simulink model "simulation"  (R2021a)
settings: Solver=VariableStepAuto  StartTime=0.0  StopTime=1  RelTol=1e-3
values from neighbouring files (symbols this model uses):
  b = 2.9e-05    [Prametre.m]
  d = 3.23e-07    [Prametre.m]
  g = 9.81    [Prametre.m]
  Ix = 0.0075    [Prametre.m]
  Iy = 0.0075    [Prametre.m]
  Iz = 0.013    [Prametre.m]
  Jr = 2.83e-05    [Prametre.m]
  K1 = 5.57e-04    (= 0.000557)    [Prametre.m]
  K2 = 5.57e-04    (= 0.000557)    [Prametre.m]
  K3 = 6.35e-04    (= 0.000635)    [Prametre.m]
  K4 = 5.57e-04    (= 0.000557)    [Prametre.m]
  K5 = 5.57e-04    (= 0.000557)    [Prametre.m]
  K6 = 6.35e-04    (= 0.000635)    [Prametre.m]
  l = 0.23    [Prametre.m]
  m = 0.65    [Prametre.m]
libraries: pid_lib x1
settings Model: Creator=dell  LastModifiedBy=Copytop
settings SolverCC: AlgebraicLoopSolver=TrustRegion
settings DataIOCC: ReturnWorkspaceOutputs=off
settings DebuggingCC: SFMachineParentedDataDiag=warning  ArithmeticOperatorsInVariantConditions=warning
settings SFSimCC: SimUseLocalCustomCode=off  CustomCodeUndefinedFunction=UseInterfaceOnly
settings RTWCC: RTWUseLocalCustomCode=off
settings CodeAppCC: StateflowObjectComments=on
settings SimscapeCC: SimscapeNormalizeSystem=off

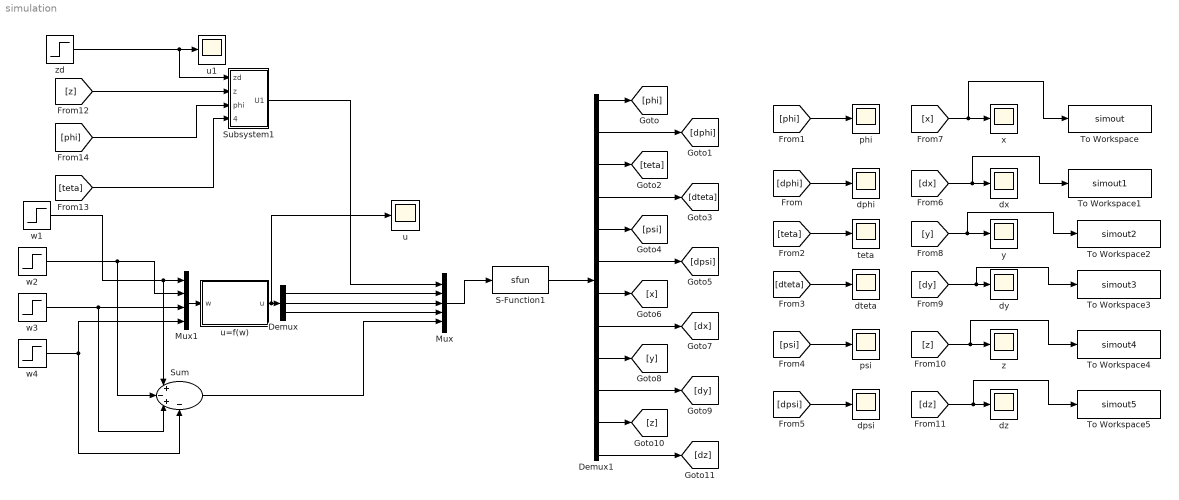
== system simulation ==
  Demux : Demux  Outputs=3
  Demux1 : Demux  Outputs=12
  Mux : Mux  Inputs=5
  Mux1 : Mux
  S-Function1 : S-Function  FunctionName=sfun  Parameters=m;l;Ix;Iy;Iz;Jr;b;d;K1;K2;K3;K4;K5;K6;g  SFunctionDeploymentMode=off  EnableBusSupport=off
  Subsystem1 : Subsystem
  Sum : Sum  Inputs=|+-+-
  To Workspace : ToWorkspace  VariableName=simout  SaveFormat=Timeseries  SampleTime=-1
  To Workspace1 : ToWorkspace  VariableName=simout1  SaveFormat=Timeseries  SampleTime=-1
  To Workspace2 : ToWorkspace  VariableName=simout2  SaveFormat=Timeseries  SampleTime=-1
  To Workspace3 : ToWorkspace  VariableName=simout3  SaveFormat=Timeseries  SampleTime=-1
  To Workspace4 : ToWorkspace  VariableName=simout4  SaveFormat=Timeseries  SampleTime=-1
  To Workspace5 : ToWorkspace  VariableName=simout5  SaveFormat=Timeseries  SampleTime=-1
  dphi : Scope
  dpsi : Scope
  dteta : Scope
  dx : Scope
  dy : Scope
  dz : Scope
  phi : Scope
  psi : Scope
  teta : Scope
  u : Scope
  u1 : Scope
  u=f(w) : MATLAB Function  TreatAsAtomicUnit=on
  w{1..4} (4 alike) : Step  Time=0  After=200  SampleTime=0
  x : Scope
  y : Scope
  z : Scope
  zd : Step  Time=0  Before=5  After=5  SampleTime=0
  wires:
  Mux/1 -> S-Function1/1
  w2/1 -> Sum/2, Mux1/2
  Mux1/1 -> u=f(w)/1(w)
  w3/1 -> Sum/3, Mux1/3
  w4/1 -> Mux1/4, Sum/4
  u=f(w)/1(u) -> u/1, Demux/1
  S-Function1/1 -> Demux1/1
  Demux1/1 -> [phi]
  Demux1/3 -> [teta]
  Demux1/5 -> [psi]
  Demux1/7 -> [x]
  Demux1/9 -> [y]
  Demux1/11 -> [z]
  [phi] -> phi/1
  [dphi] -> dphi/1
  [teta] -> teta/1
  [dteta] -> dteta/1
  [psi] -> psi/1
  [dpsi] -> dpsi/1
  [dx] -> To Workspace1/1, dx/1
  [y] -> To Workspace2/1, y/1
  [dy] -> To Workspace3/1, dy/1
  [z] -> To Workspace4/1, z/1
  [dz] -> To Workspace5/1, dz/1
  Sum/1 -> Mux/5
  Demux1/2 -> [dphi]
  Demux1/4 -> [dteta]
  Demux1/6 -> [dpsi]
  Demux1/8 -> [dx]
  Demux1/10 -> [dy]
  Demux1/12 -> [dz]
  [z] -> Subsystem1/2(z)
  [phi] -> Subsystem1/3(phi)
  zd/1 -> Subsystem1/1(zd), u1/1
  [teta] -> Subsystem1/4(teta)
  Subsystem1/1(U1) -> Mux/1
  w1/1 -> Sum/1, Mux1/1
  Demux/1 -> Mux/2
  Demux/2 -> Mux/3
  Demux/3 -> Mux/4
  [x] -> To Workspace/1, x/1

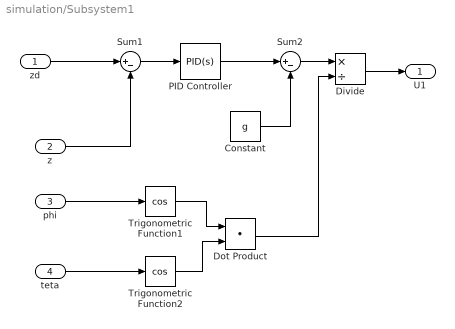
== system simulation/Subsystem1 ==
  zd : Inport
  z : Inport  Port=2
  phi : Inport  Port=3
  teta : Inport  Port=4
  Constant : Constant  Value=g
  Divide : Product  Inputs=*/
  Dot Product : DotProduct  InputSameDT=on  OutDataTypeStr=Inherit: Inherit via internal rule
  PID Controller : pid_lib/PID Controller  Controller=PID  Form=Parallel  TimeDomain=Continuous-time  UseExternalTs=off  SampleTime=-1  IntegratorMethod=Forward Euler  FilterMethod=Forward Euler  ControllerParametersSource=internal  P=100  I=0  D=42  UseFilter=on  N=100  TunerSelectOption=Transfer Function Based (PID Tuner App)  InitialConditionSource=internal  InitialConditionForIntegrator=0  InitialConditionForFilter=0  DifferentiatorICPrevScaledInput=0  ExternalReset=none  TrackingMode=off  Kt=1  LimitOutput=off  SatLimitsSource=internal  UpperSaturationLimit=inf  LowerSaturationLimit=-inf  LinearizeAsGain=on  AntiWindupMode=none  Kb=1  POutMin=[]  POutMax=[]  IOutMin=[]  IOutMax=[]  DOutMin=[]  DOutMax=[]  NOutMin=[]  NOutMax=[]  SumOutMin=[]  SumOutMax=[]  SaturationOutMin=[]  SaturationOutMax=[]  PParamMin=[]  PParamMax=[]  IParamMin=[]  IParamMax=[]  DParamMin=[]  DParamMax=[]  NParamMin=[]  NParamMax=[]  KbParamMin=[]  KbParamMax=[]  KtParamMin=[]  KtParamMax=[]  KbOutMin=[]  KbOutMax=[]  KtOutMin=[]  KtOutMax=[]  IntegratorOutMin=[]  IntegratorOutMax=[]  FilterOutMin=[]  FilterOutMax=[]  SumI1OutMin=[]  SumI1OutMax=[]  SumI2OutMin=[]  SumI2OutMax=[]  SumI3OutMin=[]  SumI3OutMax=[]  SumI4OutMin=[]  SumI4OutMax=[]  SumDOutMin=[]  SumDOutMax=[]  DifferentiatorOutMin=[]  DifferentiatorOutMax=[]  FilterDiffOutCoefMin=[]  FilterDiffOutCoefMax=[]  ReciprocalOutMin=[]  ReciprocalOutMax=[]  SumDenOutMin=[]  SumDenOutMax=[]  SumNumOutMin=[]  SumNumOutMax=[]  DivideOutMin=[]  DivideOutMax=[]  UdiffTsProdOutMin=[]  UdiffTsProdOutMax=[]  NTsProdOutMin=[]  NTsProdOutMax=[]  UintegralTsProdOutMin=[]  UintegralTsProdOutMax=[]  UngainTsProdOutMin=[]  UngainTsProdOutMax=[]  IntegratorContinuousStateAttributes=''  IntegratorStateMustResolveToSignalObject=off  IntegratorRTWStateStorageClass=Auto  FilterContinuousStateAttributes=''  FilterStateMustResolveToSignalObject=off  FilterRTWStateStorageClass=Auto  ParallelPVariant=InternalParameters  IdealPVariant=Disabled  IVariant=InternalParameters  DVariant=InternalParameters  IntegratorVariant=Continuous  SatVariant=Disabled  AWVariant=Passthrough  PCopyVariant=Disabled  TRVariant=Disabled  FdbkBlocksVariant=Forward  IdealPFdbkVariant=Disabled  SatFdbkVariant=Disabled  DerivativeFilterVariant=ContFilter  NVariant=InternalParameters  NCopyVariant=Disabled  FilterICVariant=InternalICsFilter  IntegratorICVariant=InternalICs  ExternalResetVariant=Disabled  TRSumVariant=Passthrough  SumFdbkVariant=Disabled  SumVariant=Sum_PID  TsampFilterVariant=InternalTs  TsampNgainVariant=Passthrough  TsampIntegralVariant=Passthrough  ExternalSaturationOutDataTypeStr=Inherit: Same as second input
  Sum1 : Sum  Inputs=|+-
  Sum2 : Sum  Inputs=|+-
  Trigonometric Function1 : Trigonometry  Operator=cos
  Trigonometric Function2 : Trigonometry  Operator=cos
  U1 : Outport
  wires:
  Sum1/1 -> PID Controller/1
  Sum2/1 -> Divide/1
  PID Controller/1 -> Sum2/1
  phi/1 -> Trigonometric Function1/1
  teta/1 -> Trigonometric Function2/1
  Dot Product/1 -> Divide/2
  Trigonometric Function2/1 -> Dot Product/2
  Trigonometric Function1/1 -> Dot Product/1
  Divide/1 -> U1/1
  Constant/1 -> Sum2/2
  z/1 -> Sum1/2
  zd/1 -> Sum1/1

== matlab function simulation/u=f(w) ==
  data: w input; u output
function u = fcn(w)
% w=[w1^2 w2^2 w3^2 w4^2]';
l=0.23;d=3.23e-07;
b=2.9e-05;
u =[0 -l*b 0 l*b;-l*b 0 l*b 0;d -d d -d]*[w(1)^2 w(2)^2 w(3)^2 w(4)^2]';
